simulink model "calcul_produit_2matrices"  (R2022b)
settings: Solver=VariableStepAuto  StartTime=0.0  StopTime=10.0  RelTol=1e-3
settings Model: Creator=cheye  LastModifiedBy=cheye

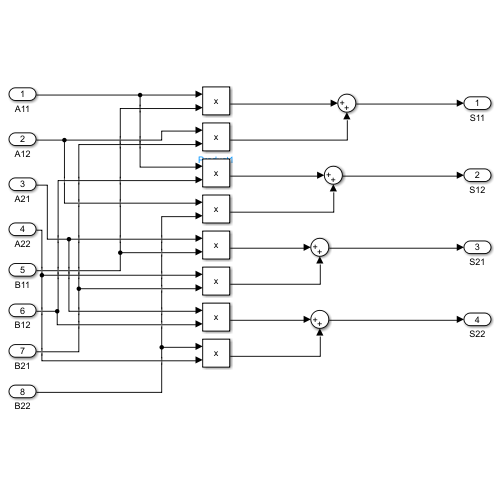
[thumbnail: Simulink's stored preview of the top-level diagram]
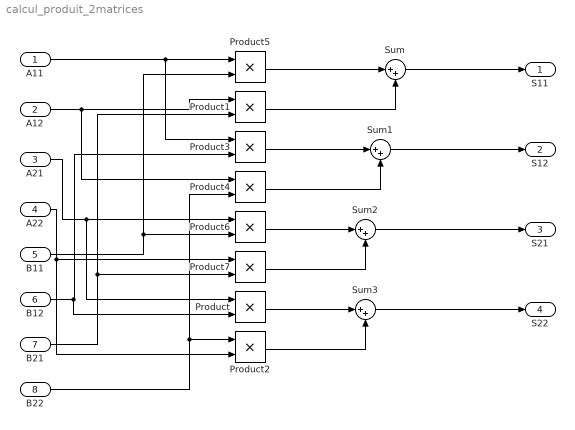
== system calcul_produit_2matrices ==
  A11 : Inport
  A12 : Inport  Port=2
  A21 : Inport  Port=3
  A22 : Inport  Port=4
  B11 : Inport  Port=5
  B12 : Inport  Port=6
  B21 : Inport  Port=7
  B22 : Inport  Port=8
  Product{,1..7} (8 alike) : Product
  Sum{,1..3} (4 alike) : Sum  Inputs=|++
  S11 : Outport
  S12 : Outport  Port=2
  S21 : Outport  Port=3
  S22 : Outport  Port=4
  wires:
  A11/1 -> Product3/1, Product5/1
  B11/1 -> Product6/2, Product5/2
  A12/1 -> Product4/1, Product1/1
  B21/1 -> Product7/2, Product1/2
  B12/1 -> Product/2, Product3/2
  B22/1 -> Product2/1, Product4/2
  A21/1 -> Product/1, Product6/1
  A22/1 -> Product2/2, Product7/1
  Product5/1 -> Sum/1
  Product1/1 -> Sum/2
  Product3/1 -> Sum1/1
  Product4/1 -> Sum1/2
  Product6/1 -> Sum2/1
  Product7/1 -> Sum2/2
  Product/1 -> Sum3/1
  Product2/1 -> Sum3/2
  Sum/1 -> S11/1
  Sum1/1 -> S12/1
  Sum2/1 -> S21/1
  Sum3/1 -> S22/1
